simulink library "lateral_model"  (R2014a)
settings: Solver=ode45  StartTime=0.0  StopTime=10.0  RelTol=1e-3
undefined symbols (not defined in the file or in its folder): par
libraries: simulink x4
settings Model: Creator=goghino  LastModifiedBy=goghino

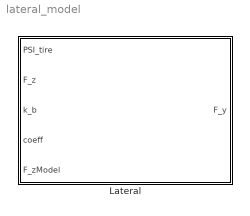
== system lateral_model ==
  Lateral : Subsystem

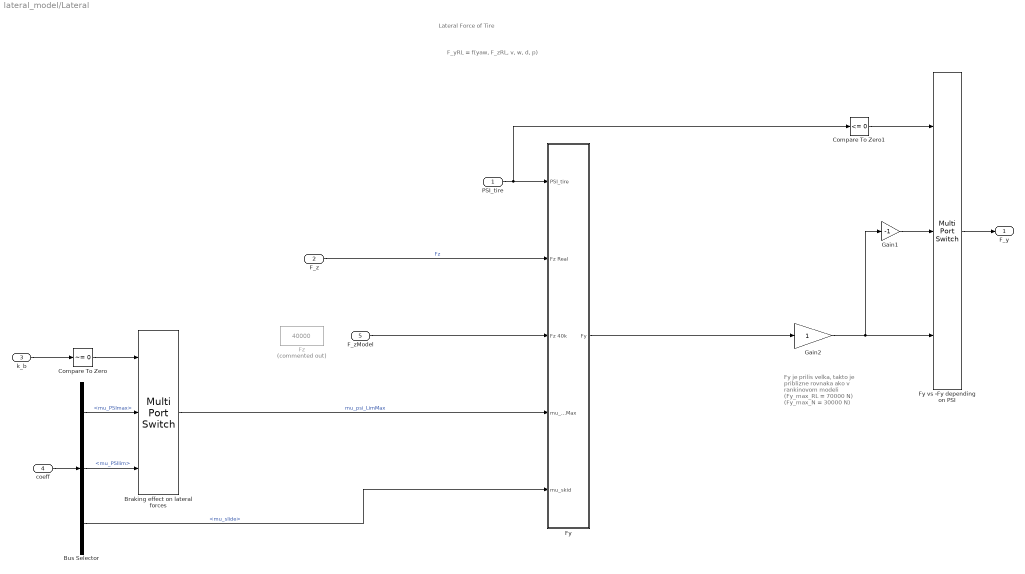
== system lateral_model/Lateral ==
  note: Fy je prilis velka,
      | takto je priblizne rovnaka
      | ako v rankinovom modeli
      | (Fy_max_RL = 70000 N)
      | (Fy_max_N = 30000 N)
  note: Lateral Force of Tire
  note: F_yRL = f(yaw, F_zRL, v, w, d, p)
  PSI_tire : Inport
  F_z : Inport  Port=2
  k_b : Inport  Port=3
  coeff : Inport  Port=4
  F_zModel : Inport  Port=5
  Braking effect on lateral forces : MultiPortSwitch  DataPortOrder=Specify indices  Inputs=2  DataPortIndices={0,1}
  Bus Selector : BusSelector  OutputSignals=mu_PSImax,mu_PSIlim,mu_slide
  Compare To Zero : simulink/Logic and Bit Operations/Compare To Zero  relop=~=  OutDataTypeStr=uint8
  Compare To Zero1 : simulink/Logic and Bit Operations/Compare To Zero  relop=<=  OutDataTypeStr=boolean
  Fy : Subsystem
  Fy vs -Fy depending on PSI : MultiPortSwitch  DataPortOrder=Specify indices  Inputs=2  DataPortIndices={0,1}
  Fz : Constant  Commented=on  Value=40000
  Gain1 : Gain  Gain=-1
  Gain2 : Gain
  F_y : Outport
  wires:
  k_b/1 -> Compare To Zero/1
  Compare To Zero/1 -> Braking effect on lateral forces/1
  Bus Selector/2 -> Braking effect on lateral forces/3  "<mu_PSIlim>"
  Bus Selector/1 -> Braking effect on lateral forces/2  "<mu_PSImax>"
  coeff/1 -> Bus Selector/1
  Fy vs -Fy depending on PSI/1 -> F_y/1
  Gain2/1 -> Gain1/1, Fy vs -Fy depending on PSI/3
  Compare To Zero1/1 -> Fy vs -Fy depending on PSI/1
  Gain1/1 -> Fy vs -Fy depending on PSI/2
  F_z/1 -> Fy/2(Fz Real)  "Fz"
  F_zModel/1 -> Fy/3(Fz 40k)
  Braking effect on lateral forces/1 -> Fy/4(mu_PSI_limMax)  "mu_psi_LimMax"
  PSI_tire/1 -> Compare To Zero1/1, Fy/1(PSI_tire)
  Bus Selector/3 -> Fy/5(mu_skid)  "<mu_slide>"
  Fy/1(Fy) -> Gain2/1

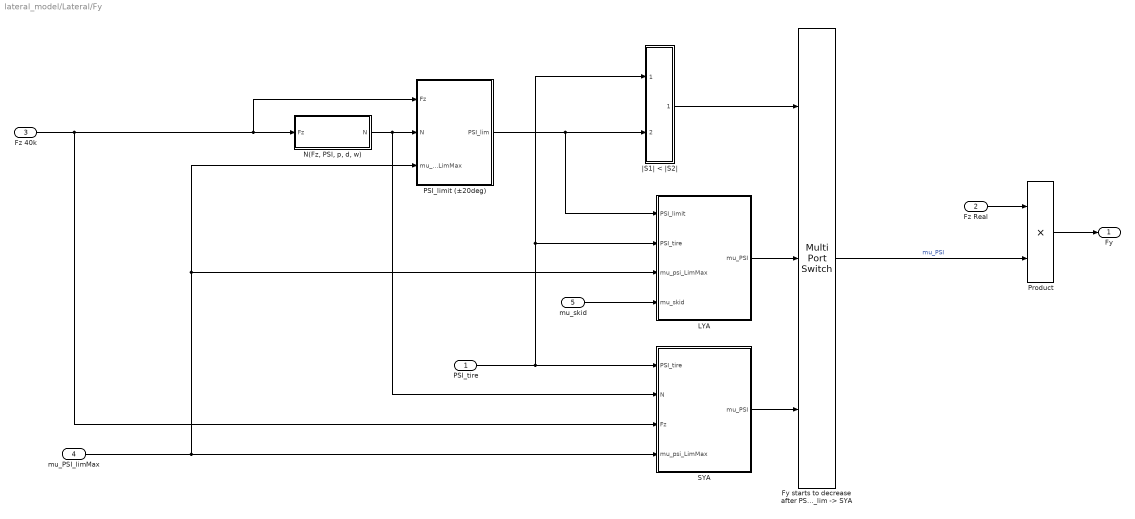
== system lateral_model/Lateral/Fy ==
  PSI_tire : Inport
  Fz Real : Inport  Port=2
  Fz 40k : Inport  Port=3
  mu_PSI_limMax : Inport  Port=4
  mu_skid : Inport  Port=5
  "Fy starts to decrease after PSI < PSI_lim -> SYA" : MultiPortSwitch  DataPortOrder=Specify indices  Inputs=2  DataPortIndices={0,1}
  LYA : Subsystem
  "N(Fz, PSI, p, d, w)" : Subsystem
  PSI_limit (±20deg) : Subsystem
  Product : Product
  SYA : Subsystem
  |S1| < |S2| : Subsystem
  Fy : Outport
  wires:
  SYA/1(mu_PSI) -> "Fy starts to decrease after PSI < PSI_lim -> SYA"/3
  Product/1 -> Fy/1
  mu_PSI_limMax/1 -> PSI_limit (±20deg)/3(mu_psi_LimMax), LYA/3(mu_psi_LimMax), SYA/4(mu_psi_LimMax)
  |S1| < |S2|/1(Out1) -> "Fy starts to decrease after PSI < PSI_lim -> SYA"/1
  PSI_limit (±20deg)/1(PSI_lim) -> |S1| < |S2|/2(S2), LYA/1(PSI_limit)
  "N(Fz, PSI, p, d, w)"/1(N) -> PSI_limit (±20deg)/2(N), SYA/2(N)
  Fz 40k/1 -> PSI_limit (±20deg)/1(Fz), "N(Fz, PSI, p, d, w)"/1(Fz), SYA/3(Fz)
  Fz Real/1 -> Product/1
  LYA/1(mu_PSI) -> "Fy starts to decrease after PSI < PSI_lim -> SYA"/2
  PSI_tire/1 -> |S1| < |S2|/1(S1), LYA/2(PSI_tire), SYA/1(PSI_tire)
  "Fy starts to decrease after PSI < PSI_lim -> SYA"/1 -> Product/2  "mu_PSI"
  mu_skid/1 -> LYA/4(mu_skid)

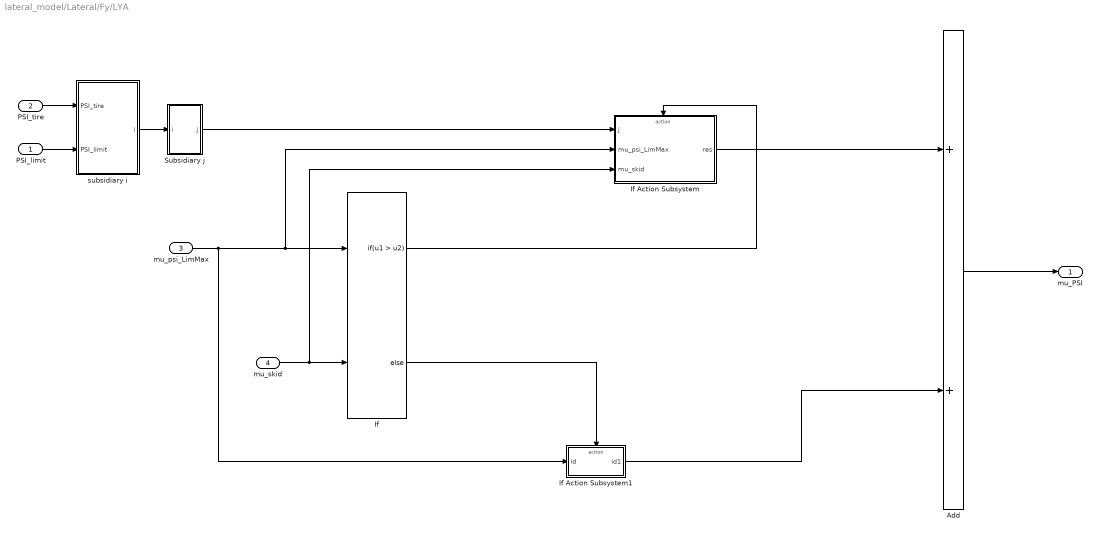
== system lateral_model/Lateral/Fy/LYA ==
  PSI_limit : Inport
  PSI_tire : Inport  Port=2
  mu_psi_LimMax : Inport  Port=3
  mu_skid : Inport  Port=4
  Add : Sum
  If : If  NumInputs=2  IfExpression=u1 > u2
  If Action Subsystem : Subsystem  TreatAsAtomicUnit=on
  If Action Subsystem1 : Subsystem  TreatAsAtomicUnit=on
  Subsidiary j : Subsystem
  subsidiary i : Subsystem
  mu_PSI : Outport
  wires:
  Subsidiary j/1(j) -> If Action Subsystem/1(j)
  mu_skid/1 -> If/2, If Action Subsystem/3(mu_skid)
  mu_psi_LimMax/1 -> If/1, If Action Subsystem/2(mu_psi_LimMax), If Action Subsystem1/1(id)
  If Action Subsystem1/1(id1) -> Add/2
  If Action Subsystem/1(res) -> Add/1
  Add/1 -> mu_PSI/1
  If/2 -> If Action Subsystem1/Action
  If/1 -> If Action Subsystem/Action
  subsidiary i/1(i) -> Subsidiary j/1(i)
  PSI_limit/1 -> subsidiary i/2(PSI_limit)
  PSI_tire/1 -> subsidiary i/1(PSI_tire)

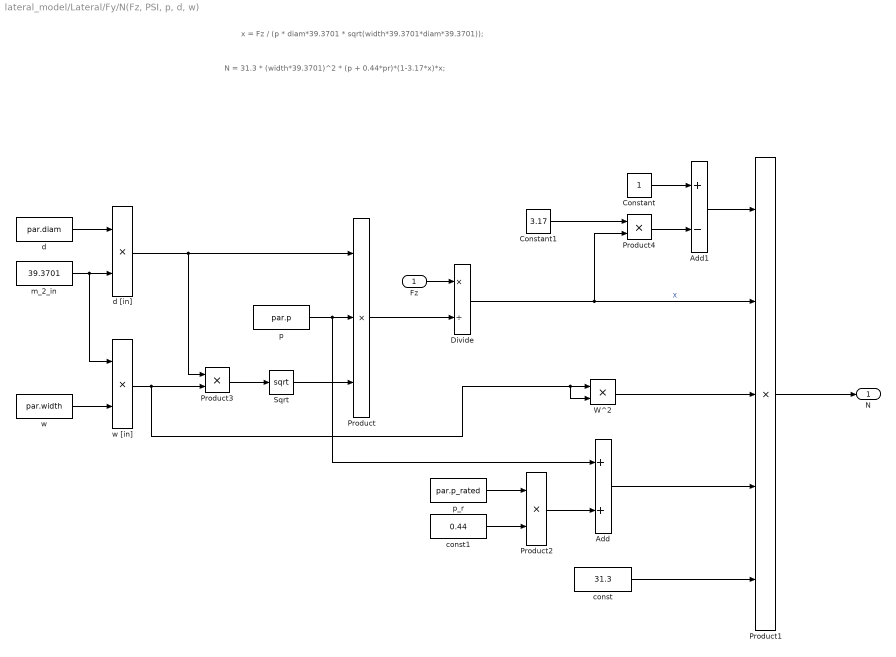
== system lateral_model/Lateral/Fy/N(Fz, PSI, p, d, w) ==
  note: x = Fz / (p * diam*39.3701 * sqrt(width*39.3701*diam*39.3701));
  note: N = 31.3 * (width*39.3701)^2 * (p + 0.44*pr)*(1-3.17*x)*x;
  Fz : Inport
  Add : Sum
  Add1 : Sum  Inputs=+-
  Constant : Constant
  Constant1 : Constant  Value=3.17
  Divide : Product  Inputs=*/
  Product : Product  Inputs=3
  Product1 : Product  Inputs=5
  Product2 : Product
  Product3 : Product
  Product4 : Product
  Sqrt : Sqrt  SaturateOnIntegerOverflow=on
  W^2 : Product
  const : Constant  Value=31.3
  "const1 " : Constant  Value=0.44
  d : Constant  Value=par.diam
  d [in] : Product
  m_2_in : Constant  Value=39.3701
  p : Constant  Value=par.p
  p_r : Constant  Value=par.p_rated
  w : Constant  Value=par.width
  w [in] : Product
  N : Outport
  wires:
  Add1/1 -> Product1/1
  Product4/1 -> Add1/2
  Constant1/1 -> Product4/1
  Constant/1 -> Add1/1
  Add/1 -> Product1/4
  Product2/1 -> Add/2
  p_r/1 -> Product2/1
  "const1 "/1 -> Product2/2
  W^2/1 -> Product1/3
  const/1 -> Product1/5
  Product1/1 -> N/1
  Divide/1 -> Product1/2, Product4/2  "X"
  Product/1 -> Divide/2
  w [in]/1 -> Product3/2, W^2/1, W^2/2
  Product3/1 -> Sqrt/1
  d [in]/1 -> Product/1, Product3/1
  w/1 -> w [in]/2
  m_2_in/1 -> d [in]/2, w [in]/1
  d/1 -> d [in]/1
  Sqrt/1 -> Product/3
  p/1 -> Product/2, Add/1
  Fz/1 -> Divide/1

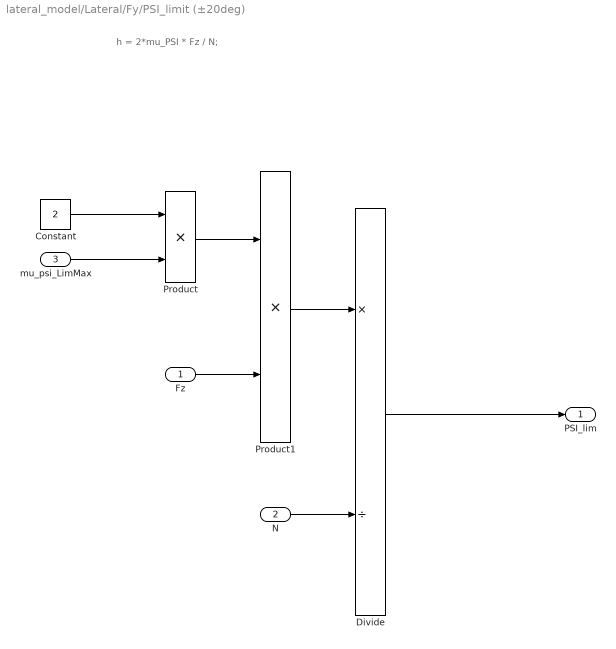
== system lateral_model/Lateral/Fy/PSI_limit (±20deg) ==
  note: h = 2*mu_PSI * Fz / N;
  Fz : Inport
  N : Inport  Port=2
  mu_psi_LimMax : Inport  Port=3
  Constant : Constant  Value=2
  Divide : Product  Inputs=*/
  Product : Product
  Product1 : Product
  PSI_lim : Outport
  wires:
  Divide/1 -> PSI_lim/1
  N/1 -> Divide/2
  Product1/1 -> Divide/1
  Fz/1 -> Product1/2
  Product/1 -> Product1/1
  mu_psi_LimMax/1 -> Product/2
  Constant/1 -> Product/1

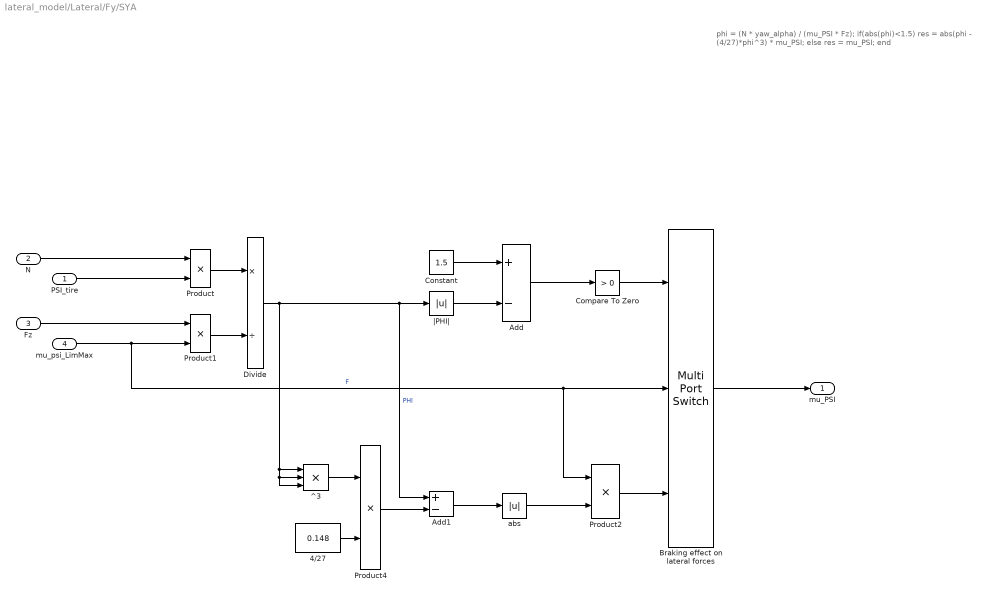
== system lateral_model/Lateral/Fy/SYA ==
  note: phi = (N * yaw_alpha) / (mu_PSI * Fz);
      | if(abs(phi)<1.5)
      | res = abs(phi - (4/27)*phi^3) * mu_PSI;
      | else
      | res = mu_PSI;
      | end
  PSI_tire : Inport
  N : Inport  Port=2
  Fz : Inport  Port=3
  mu_psi_LimMax : Inport  Port=4
  4/27 : Constant  Value=0.148
  Add : Sum  Inputs=+-
  Add1 : Sum  Inputs=+-
  Braking effect on lateral forces : MultiPortSwitch  DataPortOrder=Specify indices  Inputs=2  DataPortIndices={0,1}
  Compare To Zero : simulink/Logic and Bit Operations/Compare To Zero  relop=>  OutDataTypeStr=boolean
  Constant : Constant  Value=1.5
  Divide : Product  Inputs=*/
  Product{,1..2,4} (4 alike) : Product
  ^3 : Product  Inputs=3
  abs : Abs
  |PHI| : Abs
  mu_PSI : Outport
  wires:
  ^3/1 -> Product4/1
  4/27/1 -> Product4/2
  Product4/1 -> Add1/2
  Add1/1 -> abs/1
  abs/1 -> Product2/2
  Product2/1 -> Braking effect on lateral forces/3
  mu_psi_LimMax/1 -> Product1/2, Braking effect on lateral forces/2, Product2/1  "F"
  Braking effect on lateral forces/1 -> mu_PSI/1
  Compare To Zero/1 -> Braking effect on lateral forces/1
  Add/1 -> Compare To Zero/1
  |PHI|/1 -> Add/2
  Constant/1 -> Add/1
  Divide/1 -> |PHI|/1, Add1/1, ^3/3, ^3/2, ^3/1  "PHI"
  Product1/1 -> Divide/2
  Product/1 -> Divide/1
  Fz/1 -> Product1/1
  PSI_tire/1 -> Product/2
  N/1 -> Product/1

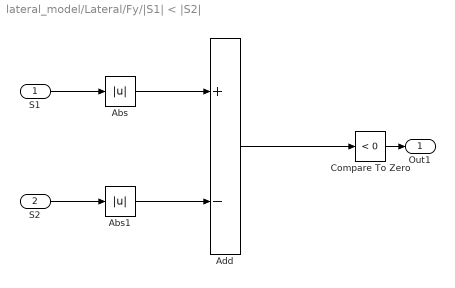
== system lateral_model/Lateral/Fy/|S1| < |S2| ==
  S1 : Inport
  S2 : Inport  Port=2
  Abs : Abs
  Abs1 : Abs
  Add : Sum  Inputs=+-
  Compare To Zero : simulink/Logic and Bit Operations/Compare To Zero  relop=<  OutDataTypeStr=uint8
  Out1 : Outport
  wires:
  Add/1 -> Compare To Zero/1
  Abs1/1 -> Add/2
  Abs/1 -> Add/1
  S1/1 -> Abs/1
  S2/1 -> Abs1/1
  Compare To Zero/1 -> Out1/1

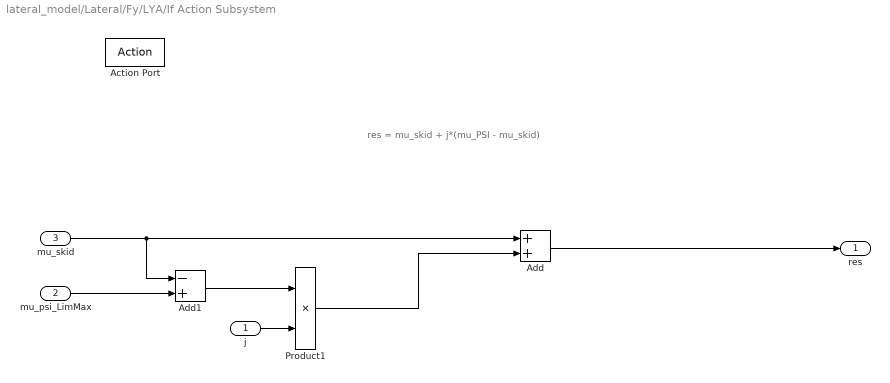
== system lateral_model/Lateral/Fy/LYA/If Action Subsystem ==
  note: res = mu_skid + j*(mu_PSI - mu_skid)
  j : Inport
  mu_psi_LimMax : Inport  Port=2
  mu_skid : Inport  Port=3
  Action Port : ActionPort  InitializeStates=reset  PropagateVarSize=During execution
  Add : Sum
  Add1 : Sum  Inputs=-+
  Product1 : Product
  res : Outport  OutputWhenDisabled=reset  InitialOutput=[0]
  wires:
  mu_psi_LimMax/1 -> Add1/2
  Add1/1 -> Product1/1
  mu_skid/1 -> Add/1, Add1/1
  Add/1 -> res/1
  Product1/1 -> Add/2
  j/1 -> Product1/2

== system lateral_model/Lateral/Fy/LYA/If Action Subsystem1 ==
  id : Inport
  Action Port : ActionPort  InitializeStates=reset
  id1 : Outport  OutputWhenDisabled=reset  InitialOutput=[0]
  wires:
  id/1 -> id1/1

== system lateral_model/Lateral/Fy/LYA/Subsidiary j ==
  i : Inport
  Add : Sum
  If : If  IfExpression=u1 < 0.3
  If Action Subsystem : Subsystem  TreatAsAtomicUnit=on
  If Action Subsystem1 : Subsystem  TreatAsAtomicUnit=on
  j : Outport
  wires:
  If Action Subsystem1/1(j) -> Add/2
  If Action Subsystem/1(j) -> Add/1
  Add/1 -> j/1
  If/2 -> If Action Subsystem1/Action
  If/1 -> If Action Subsystem/Action
  i/1 -> If Action Subsystem/1(i), If Action Subsystem1/1(i), If/1

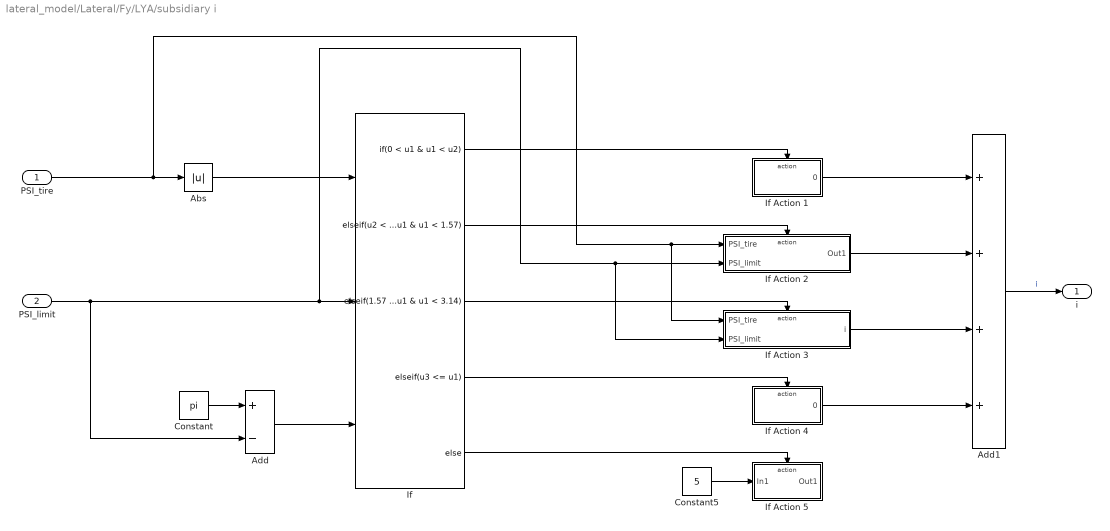
== system lateral_model/Lateral/Fy/LYA/subsidiary i ==
  PSI_tire : Inport
  PSI_limit : Inport  Port=2
  Abs : Abs
  Add : Sum  Inputs=+-
  Add1 : Sum  Inputs=++++
  Constant : Constant  Value=pi
  Constant5 : Constant  Value=5
  If : If  NumInputs=3  IfExpression=0 < u1 & u1 < u2  ElseIfExpressions="u2 <  u1 & u1 < 1.57, 1.57 < u1 & u1 < 3.14, u3 <= u1"
  If Action 1 : Subsystem  TreatAsAtomicUnit=on
  If Action 2 : Subsystem  TreatAsAtomicUnit=on
  If Action 3 : Subsystem  TreatAsAtomicUnit=on
  If Action 4 : Subsystem  TreatAsAtomicUnit=on
  If Action 5 : Subsystem  TreatAsAtomicUnit=on
  i : Outport
  wires:
  Constant/1 -> Add/1
  PSI_limit/1 -> Add/2, If/2, If Action 2/2(PSI_limit), If Action 3/2(PSI_limit)
  If Action 1/1(0) -> Add1/1
  If Action 4/1(0) -> Add1/4
  Constant5/1 -> If Action 5/1(In1)
  Add1/1 -> i/1  "i"
  If Action 2/1(Out1) -> Add1/2
  If/3 -> If Action 3/Action
  If/5 -> If Action 5/Action
  Abs/1 -> If/1
  Add/1 -> If/3
  If/2 -> If Action 2/Action
  If/1 -> If Action 1/Action
  If/4 -> If Action 4/Action
  If Action 3/1(i) -> Add1/3
  PSI_tire/1 -> Abs/1, If Action 2/1(PSI_tire), If Action 3/1(PSI_tire)

== system lateral_model/Lateral/Fy/LYA/Subsidiary j/If Action Subsystem ==
  note: j = 1 - 1.93*i;
  i : Inport
  Action Port : ActionPort  InitializeStates=reset  PropagateVarSize=During execution
  Add : Sum  Inputs=+-
  Constant : Constant
  Constant1 : Constant  Value=1.93
  Product1 : Product
  j : Outport  OutputWhenDisabled=reset  InitialOutput=[0]
  wires:
  Add/1 -> j/1
  Product1/1 -> Add/2
  i/1 -> Product1/1
  Constant1/1 -> Product1/2
  Constant/1 -> Add/1

== system lateral_model/Lateral/Fy/LYA/Subsidiary j/If Action Subsystem1 ==
  note: j = 0.58 - 0.575*i;
  i : Inport
  Action Port : ActionPort  InitializeStates=reset
  Add : Sum  Inputs=+-
  Constant : Constant  Value=0.58
  Constant1 : Constant  Value=0.575
  Product1 : Product
  j : Outport  OutputWhenDisabled=reset  InitialOutput=[0]
  wires:
  Add/1 -> j/1
  Product1/1 -> Add/2
  i/1 -> Product1/1
  Constant1/1 -> Product1/2
  Constant/1 -> Add/1

== system lateral_model/Lateral/Fy/LYA/subsidiary i/If Action 1 ==
  Action Port : ActionPort  InitializeStates=reset  PropagateVarSize=During execution
  Constant1 : Constant  Value=0
  0 : Outport  OutputWhenDisabled=reset  InitialOutput=[0]
  wires:
  Constant1/1 -> 0/1

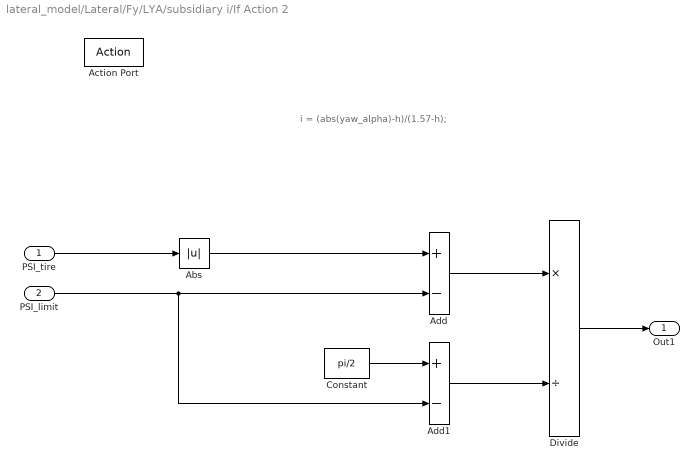
== system lateral_model/Lateral/Fy/LYA/subsidiary i/If Action 2 ==
  note: i = (abs(yaw_alpha)-h)/(1.57-h);
  PSI_tire : Inport
  PSI_limit : Inport  Port=2
  Action Port : ActionPort  InitializeStates=reset
  Abs : Abs
  Add : Sum  Inputs=+-
  Add1 : Sum  Inputs=+-
  Constant : Constant  Value=pi/2
  Divide : Product  Inputs=*/
  Out1 : Outport  OutputWhenDisabled=reset  InitialOutput=[0]
  wires:
  Abs/1 -> Add/1
  PSI_tire/1 -> Abs/1
  PSI_limit/1 -> Add/2, Add1/2
  Constant/1 -> Add1/1
  Add1/1 -> Divide/2
  Add/1 -> Divide/1
  Divide/1 -> Out1/1

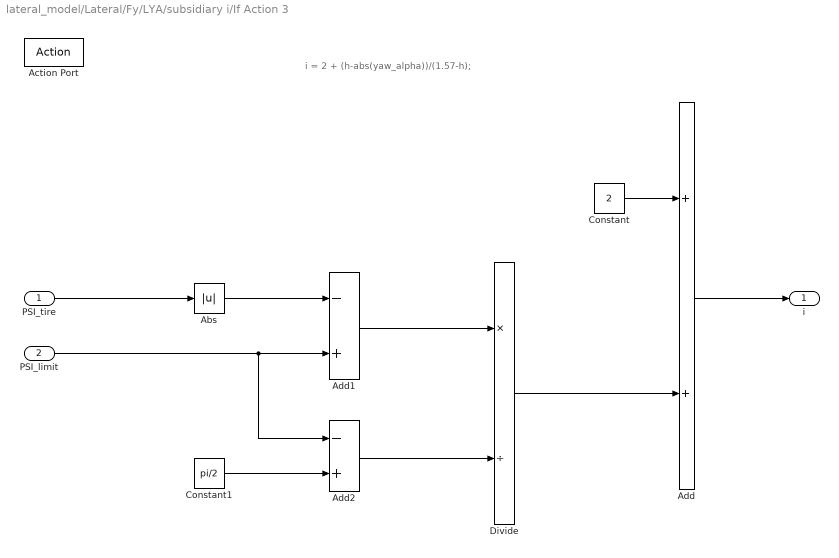
== system lateral_model/Lateral/Fy/LYA/subsidiary i/If Action 3 ==
  note: i = 2 + (h-abs(yaw_alpha))/(1.57-h);
  PSI_tire : Inport
  PSI_limit : Inport  Port=2
  Action Port : ActionPort  InitializeStates=reset  PropagateVarSize=During execution
  Abs : Abs
  Add : Sum
  Add1 : Sum  Inputs=-+
  Add2 : Sum  Inputs=-+
  Constant : Constant  Value=2
  Constant1 : Constant  Value=pi/2
  Divide : Product  Inputs=*/
  i : Outport  OutputWhenDisabled=reset  InitialOutput=[0]
  wires:
  Add/1 -> i/1
  Divide/1 -> Add/2
  Constant1/1 -> Add2/2
  Add2/1 -> Divide/2
  Add1/1 -> Divide/1
  PSI_limit/1 -> Add1/2, Add2/1
  Abs/1 -> Add1/1
  PSI_tire/1 -> Abs/1
  Constant/1 -> Add/1

== system lateral_model/Lateral/Fy/LYA/subsidiary i/If Action 4 ==
  Action Port : ActionPort  InitializeStates=reset  PropagateVarSize=During execution
  Constant1 : Constant  Value=0
  0 : Outport  OutputWhenDisabled=reset  InitialOutput=[0]
  wires:
  Constant1/1 -> 0/1

== system lateral_model/Lateral/Fy/LYA/subsidiary i/If Action 5 ==
  In1 : Inport
  Action Port : ActionPort  InitializeStates=reset  PropagateVarSize=During execution
  Out1 : Outport  OutputWhenDisabled=reset  InitialOutput=[0]
  wires:
  In1/1 -> Out1/1
